simulink model "Example_PHEX"  (R2017a)
settings: Solver=VariableStepAuto  StartTime=0.0  StopTime=10.0  RelTol=1e-3
values from neighbouring files (symbols this model uses):
  L = [0.519243383422 0.571231761788 0.460093985593 1.39194595515 0.630156881592 0.260948993381 9.53677639553 0.00918592125768 0.177711077409 0.0643194958333 0.141274848846 0.223226056913 ... (18 elements, 9x2)]    [Example_PHEX.mat]
  u0 = [60 10 0.25 0.15]    [Example_PHEX.mat]
  x0 = [54.5367745473 47.8290809093 39.5934416646 44.0109305589 34.9055548044 23.7260654078 44.0109305589 39.5934416646 39.5934416646]    [Example_PHEX.mat]
  y0 = [44.0109305589 39.5934416646]    [Example_PHEX.mat]
undefined symbols (not defined in the file or in its folder): PHEX_sys_bilin
settings Model: Creator=lerch  LastModifiedBy=lerch
settings OptimizationCC: DefaultParameterBehavior=Inlined

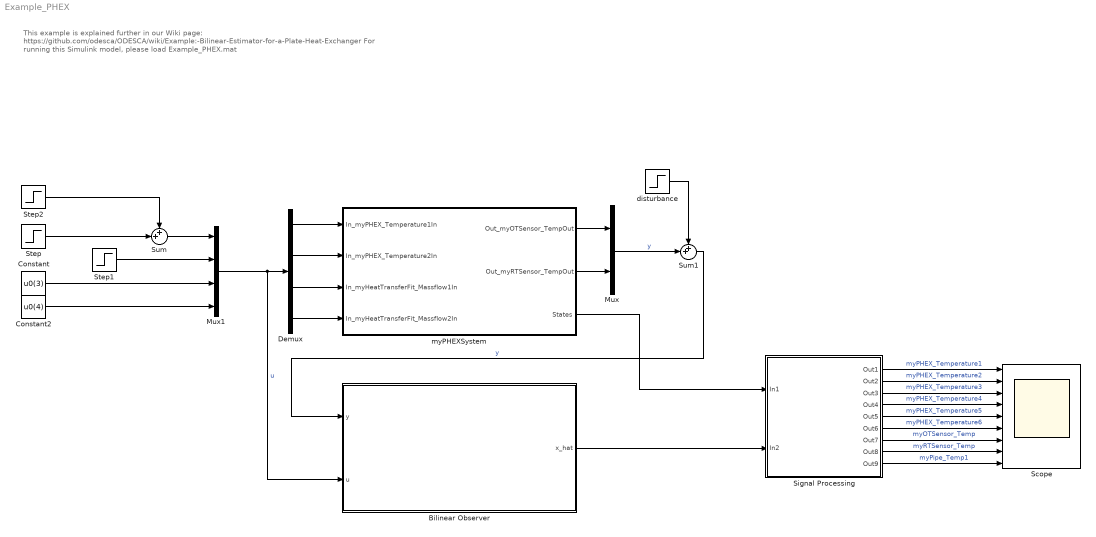
== system Example_PHEX ==
  note: This example is explained further in our Wiki page:
      | https://github.com/odesca/ODESCA/wiki/Example:-Bilinear-Estimator-for-a-Plate-Heat-Exchanger
      |
      | For running this Simulink model, please load Example_PHEX.mat
  Bilinear Observer : Subsystem
  Constant : Constant  Value=u0(3)
  Constant2 : Constant  Value=u0(4)
  Demux : Demux
  Mux : Mux  Inputs=2
  Mux1 : Mux
  Scope : Scope  NumInputPorts=9
  Signal Processing : Subsystem
  Step : Step  Before=u0(1)  After=u0(1)+20  SampleTime=0
  Step1 : Step  Time=3  Before=u0(2)  After=u0(2)+20  SampleTime=0
  Step2 : Step  Time=5  After=-40  SampleTime=0
  Sum : Sum  Inputs=++|
  Sum1 : Sum  Inputs=++|
  disturbance : Step  Time=7  After=5  SampleTime=0
  myPHEXSystem : Subsystem  mask(myPHEXSystem){initState=[0,0,0,0,0,0,0,0,0], myPHEX_cHex=500, myPHEX_mHex=1.154, myPHEX_Volume1=0.000216, myPHEX_Volume2=0.00024, myPHEX_HexArea=0.216, myPHEX_RhoFluid=998, myPHEX_cFluid=4182, myHeatTransferFit_c1=6529, myHeatTransferFit_c2=4029, myHeatTransferFit_c3=3.29, myOTSensor_TimeConst=1.8, myOTSensor_Gain=1, myPipe_cPipe=1, myPipe_mPipe=150, myPipe_VPipe=0.00055}
      mask prompts: initState "Initial State is a column vector of 9 elements:

x1 = myPHEX_Temperature1 [°C]
x2 = myPHEX_Temperature2 [°C]
x3 = myPHEX_Temperature3 [°C]
x4 = myPHEX_Temperature4 [°C]
x5 = myPHEX_Temperature5 [°C]
x6 = myPHEX_Temperature6 [°C]
x7 = myOTSensor_Temp [°C]
x8 = myRTSensor_Temp [°C]
x9 = myPipe_Temp1 [°C]

Initial State:"; myPHEX_cHex "cHex
[J/kg*K]"; myPHEX_mHex "mHex
[kg]"; myPHEX_Volume1 "Volume1
[m^3]"; myPHEX_Volume2 "Volume2
[m^3]"; myPHEX_HexArea "HexArea
[m^2]"; myPHEX_RhoFluid "RhoFluid
[kg/m^3]"; myPHEX_cFluid "cFluid
[J/kg*K]"; myHeatTransferFit_c1 "c1
[W/m^2*K)]"; myHeatTransferFit_c2 "c2
[W*s/m^2*K*kg]"; myHeatTransferFit_c3 "c3
[W*s/m^2*K*kg]"; myOTSensor_TimeConst "TimeConst
[s]"; myOTSensor_Gain "Gain
[1]"; myPipe_cPipe "cPipe
[J/kg*K]"; myPipe_mPipe "mPipe
[kg]"; myPipe_VPipe "VPipe
[m^3]"
      mask help:
      | This system consists of:
      |
      | 5 Components
      | 9 States
      | 4 Inputs
      | 2 Outputs
      | 15 Parameters
  wires:
  myPHEXSystem/1(Out_myOTSensor_TempOut) -> Mux/1
  myPHEXSystem/2(Out_myRTSensor_TempOut) -> Mux/2
  Sum1/1 -> Bilinear Observer/1(y)  "y"
  Demux/1 -> myPHEXSystem/1(In_myPHEX_Temperature1In)
  Demux/3 -> myPHEXSystem/3(In_myHeatTransferFit_Massflow1In)
  Demux/2 -> myPHEXSystem/2(In_myPHEX_Temperature2In)
  Demux/4 -> myPHEXSystem/4(In_myHeatTransferFit_Massflow2In)
  Mux1/1 -> Bilinear Observer/2(u), Demux/1  "u"
  myPHEXSystem/3(States) -> Signal Processing/1(In1)
  Bilinear Observer/1(x_hat) -> Signal Processing/2(In2)
  Signal Processing/1(Out1) -> Scope/1  "myPHEX_Temperature1"
  Signal Processing/2(Out2) -> Scope/2  "myPHEX_Temperature2"
  Signal Processing/3(Out3) -> Scope/3  "myPHEX_Temperature3"
  Signal Processing/4(Out4) -> Scope/4  "myPHEX_Temperature4"
  Signal Processing/5(Out5) -> Scope/5  "myPHEX_Temperature5"
  Signal Processing/6(Out6) -> Scope/6  "myPHEX_Temperature6"
  Signal Processing/7(Out7) -> Scope/7  "myOTSensor_Temp"
  Signal Processing/8(Out8) -> Scope/8  "myRTSensor_Temp"
  Signal Processing/9(Out9) -> Scope/9  "myPipe_Temp1"
  Step/1 -> Sum/2
  Step1/1 -> Mux1/2
  Constant/1 -> Mux1/3
  Constant2/1 -> Mux1/4
  Sum/1 -> Mux1/1
  Step2/1 -> Sum/1
  Mux/1 -> Sum1/2  "y"
  disturbance/1 -> Sum1/1

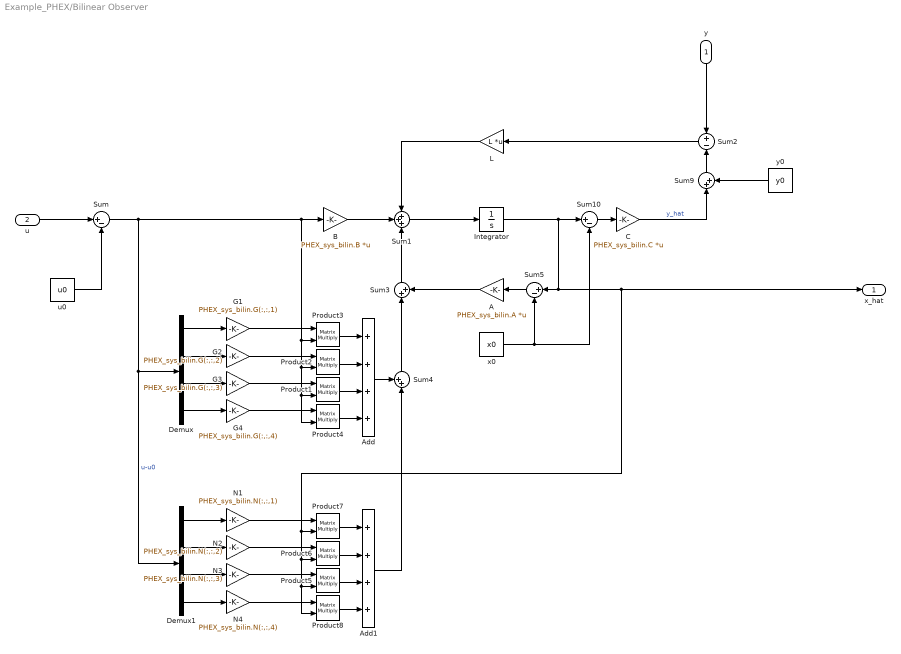
== system Example_PHEX/Bilinear Observer ==
  y : Inport
  u : Inport  Port=2
  A : Gain  Gain=PHEX_sys_bilin.A  Multiplication=Matrix(K*u) (u vector)
  Add : Sum  Inputs=++++
  Add1 : Sum  Inputs=++++
  B : Gain  Gain=PHEX_sys_bilin.B  Multiplication=Matrix(K*u) (u vector)
  C : Gain  Gain=PHEX_sys_bilin.C  Multiplication=Matrix(K*u) (u vector)
  Demux : Demux
  Demux1 : Demux
  G1 : Gain  Gain=PHEX_sys_bilin.G(:,:,1)
  G2 : Gain  Gain=PHEX_sys_bilin.G(:,:,2)
  G3 : Gain  Gain=PHEX_sys_bilin.G(:,:,3)
  G4 : Gain  Gain=PHEX_sys_bilin.G(:,:,4)
  Integrator : Integrator
  L : Gain  Gain=L  Multiplication=Matrix(K*u) (u vector)
  N1 : Gain  Gain=PHEX_sys_bilin.N(:,:,1)
  N2 : Gain  Gain=PHEX_sys_bilin.N(:,:,2)
  N3 : Gain  Gain=PHEX_sys_bilin.N(:,:,3)
  N4 : Gain  Gain=PHEX_sys_bilin.N(:,:,4)
  Product{1..8} (8 alike) : Product  Multiplication=Matrix(*)
  Sum : Sum  Inputs=|+-
  Sum1 : Sum  Inputs=+++
  Sum10 : Sum  Inputs=|+-
  Sum2 : Sum  Inputs=+-
  Sum3 : Sum  Inputs=|++
  Sum4 : Sum  Inputs=++|
  Sum5 : Sum  Inputs=|+-
  Sum9 : Sum  Inputs=|++
  u0 : Constant  Value=u0
  x0 : Constant  Value=x0
  "y0 " : Constant  Value=y0
  x_hat : Outport
  wires:
  u/1 -> Sum/1
  u0/1 -> Sum/2
  B/1 -> Sum1/2
  Sum1/1 -> Integrator/1
  C/1 -> Sum9/1  "y_hat"
  L/1 -> Sum1/1
  Sum2/1 -> L/1
  Sum5/1 -> A/1
  x0/1 -> Sum5/2, Sum10/2
  Sum10/1 -> C/1
  y/1 -> Sum2/1
  Sum9/1 -> Sum2/2
  "y0 "/1 -> Sum9/2
  Sum3/1 -> Sum1/3
  A/1 -> Sum3/2
  Demux/1 -> G1/1
  Demux/2 -> G2/1
  Demux/3 -> G3/1
  Demux/4 -> G4/1
  G1/1 -> Product3/1
  G2/1 -> Product2/1
  G3/1 -> Product1/1
  G4/1 -> Product4/1
  Product3/1 -> Add/1
  Product2/1 -> Add/2
  Product1/1 -> Add/3
  Product4/1 -> Add/4
  Add/1 -> Sum4/1
  Sum4/1 -> Sum3/1
  Add1/1 -> Sum4/2
  Product8/1 -> Add1/4
  Product5/1 -> Add1/3
  Product6/1 -> Add1/2
  Product7/1 -> Add1/1
  N4/1 -> Product8/1
  N3/1 -> Product5/1
  N2/1 -> Product6/1
  N1/1 -> Product7/1
  Demux1/4 -> N4/1
  Demux1/3 -> N3/1
  Demux1/2 -> N2/1
  Demux1/1 -> N1/1
  Integrator/1 -> Sum10/1, Sum5/1, Product7/2, Product6/2, Product5/2, Product8/2, x_hat/1
  Sum/1 -> Demux1/1, Demux/1, Product4/2, Product1/2, Product2/2, Product3/2, B/1  "u-u0"

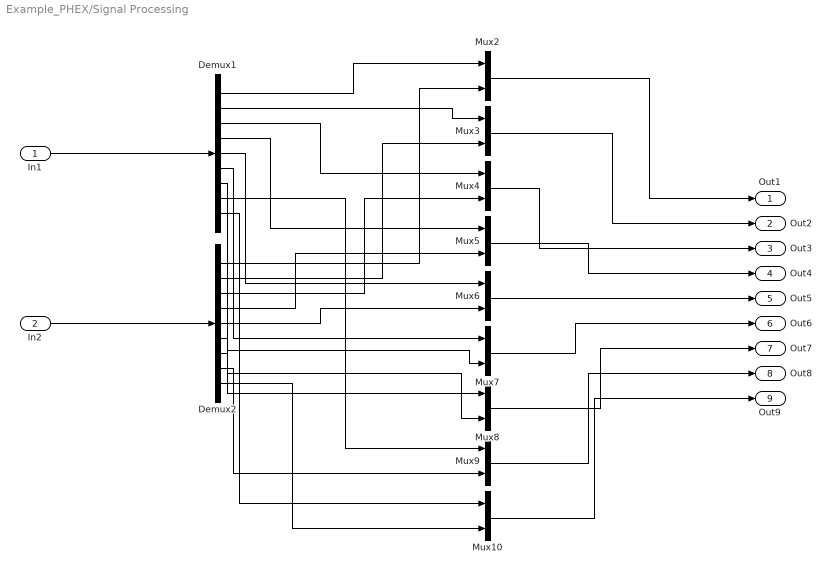
== system Example_PHEX/Signal Processing ==
  In1 : Inport
  In2 : Inport  Port=2
  Demux1 : Demux  Outputs=9
  Demux2 : Demux  Outputs=9
  Mux{2..10} (9 alike) : Mux  Inputs=2
  Out1 : Outport
  Out2 : Outport  Port=2
  Out3 : Outport  Port=3
  Out4 : Outport  Port=4
  Out5 : Outport  Port=5
  Out6 : Outport  Port=6
  Out7 : Outport  Port=7
  Out8 : Outport  Port=8
  Out9 : Outport  Port=9
  wires:
  Demux1/6 -> Mux7/1
  Demux1/4 -> Mux5/1
  In2/1 -> Demux2/1
  Demux2/8 -> Mux9/2
  Demux1/9 -> Mux10/1
  Demux1/8 -> Mux9/1
  Demux2/1 -> Mux2/2
  Demux1/7 -> Mux8/1
  Demux1/2 -> Mux3/1
  Demux1/3 -> Mux4/1
  Demux1/1 -> Mux2/1
  In1/1 -> Demux1/1
  Demux2/4 -> Mux5/2
  Mux7/1 -> Out6/1
  Demux1/5 -> Mux6/1
  Demux2/2 -> Mux3/2
  Demux2/7 -> Mux8/2
  Demux2/5 -> Mux6/2
  Demux2/9 -> Mux10/2
  Demux2/6 -> Mux7/2
  Demux2/3 -> Mux4/2
  Mux2/1 -> Out1/1
  Mux3/1 -> Out2/1
  Mux5/1 -> Out4/1
  Mux6/1 -> Out5/1
  Mux4/1 -> Out3/1
  Mux10/1 -> Out9/1
  Mux8/1 -> Out7/1
  Mux9/1 -> Out8/1

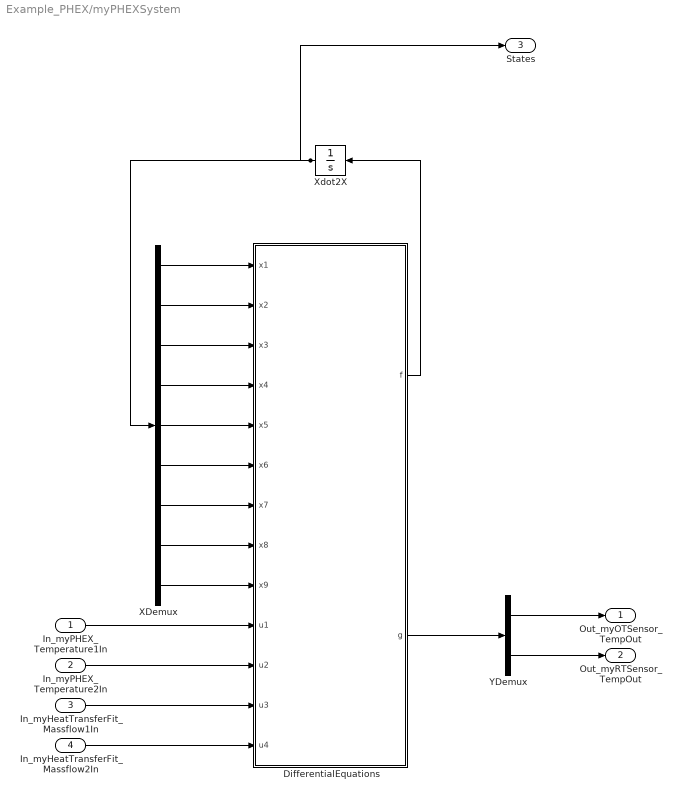
== system Example_PHEX/myPHEXSystem ==
  In_myPHEX_Temperature1In : Inport
  In_myPHEX_Temperature2In : Inport  Port=2
  In_myHeatTransferFit_Massflow1In : Inport  Port=3
  In_myHeatTransferFit_Massflow2In : Inport  Port=4
  DifferentialEquations : MATLAB Function  TreatAsAtomicUnit=on
  XDemux : Demux  Outputs=9
  Xdot2X : Integrator  InitialCondition=initState
  YDemux : Demux  Outputs=2
  Out_myOTSensor_TempOut : Outport
  Out_myRTSensor_TempOut : Outport  Port=2
  States : Outport  Port=3
  wires:
  In_myPHEX_Temperature1In/1 -> DifferentialEquations/10(u1)
  In_myPHEX_Temperature2In/1 -> DifferentialEquations/11(u2)
  In_myHeatTransferFit_Massflow1In/1 -> DifferentialEquations/12(u3)
  In_myHeatTransferFit_Massflow2In/1 -> DifferentialEquations/13(u4)
  DifferentialEquations/2(g) -> YDemux/1
  YDemux/1 -> Out_myOTSensor_TempOut/1
  YDemux/2 -> Out_myRTSensor_TempOut/1
  XDemux/1 -> DifferentialEquations/1(x1)
  XDemux/2 -> DifferentialEquations/2(x2)
  XDemux/3 -> DifferentialEquations/3(x3)
  XDemux/4 -> DifferentialEquations/4(x4)
  XDemux/5 -> DifferentialEquations/5(x5)
  XDemux/6 -> DifferentialEquations/6(x6)
  XDemux/7 -> DifferentialEquations/7(x7)
  XDemux/8 -> DifferentialEquations/8(x8)
  XDemux/9 -> DifferentialEquations/9(x9)
  DifferentialEquations/1(f) -> Xdot2X/1
  Xdot2X/1 -> XDemux/1, States/1

== matlab function Example_PHEX/myPHEXSystem/DifferentialEquations ==
  data: x1 input; f output; x2 input; x3 input; x4 input; x5 input; x6 input; x7 input; x8 input; x9 input; u1 input; u2 input; u3 input; u4 input; g output; myPipe_VPipe parameter; myPipe_mPipe parameter; myPipe_cPipe parameter; myOTSensor_Gain parameter; myOTSensor_TimeConst parameter; myHeatTransferFit_c3 parameter; myHeatTransferFit_c2 parameter; myHeatTransferFit_c1 parameter; myPHEX_cFluid parameter; myPHEX_RhoFluid parameter; myPHEX_HexArea parameter; myPHEX_Volume2 parameter; myPHEX_Volume1 parameter; myPHEX_mHex parameter; myPHEX_cHex parameter
function [f,g] = DifferentialEquations(x1,x2,x3,x4,x5,x6,x7,x8,x9,u1,u2,u3,u4,myPipe_VPipe, myPipe_mPipe, myPipe_cPipe, myOTSensor_Gain, myOTSensor_TimeConst, myHeatTransferFit_c3, myHeatTransferFit_c2, myHeatTransferFit_c1, myPHEX_cFluid, myPHEX_RhoFluid, myPHEX_HexArea, myPHEX_Volume2, myPHEX_Volume1, myPHEX_mHex, myPHEX_cHex)
%#codegen

%    This function was generated by the Symbolic Math Toolbox version 7.2.
%    02-Jul-2019 09:48:33

t2 = myHeatTransferFit_c2.*u3;
t3 = myHeatTransferFit_c3.*u4;
t4 = myHeatTransferFit_c1+t2+t3;
t5 = myPHEX_cHex.*myPHEX_mHex.*(1.0./6.0);
t6 = myPHEX_cFluid.*myPHEX_Volume1.*myPHEX_RhoFluid.*(1.0./3.0);
t7 = t5+t6;
t8 = 1.0./t7;
t9 = x1-x4;
t10 = myPHEX_HexArea.*t4.*t9.*(1.0./3.0);
t11 = x2-x5;
t12 = myPHEX_HexArea.*t4.*t11.*(1.0./3.0);
t13 = myPHEX_cFluid.*myPHEX_Volume2.*myPHEX_RhoFluid.*(1.0./3.0);
t14 = t5+t13;
t15 = 1.0./t14;
t16 = x3-x6;
t17 = myPHEX_HexArea.*t4.*t16.*(1.0./3.0);
t18 = 1.0./myOTSensor_TimeConst;
f = [-t8.*(t10-myPHEX_cFluid.*u3.*(u1-x1));-t8.*(t12-myPHEX_cFluid.*u3.*(x1-x2));-t8.*(t17-myPHEX_cFluid.*u3.*(x2-x3));t15.*(t10-myPHEX_cFluid.*u4.*(x4-x5));t15.*(t12-myPHEX_cFluid.*u4.*(x5-x6));t15.*(t17+myPHEX_cFluid.*u4.*(u2-x6));-t18.*(x7-myOTSensor_Gain.*x4);-t18.*(x8-myOTSensor_Gain.*x9);(myPHEX_cFluid.*u3.*(x3-x9))./(myPipe_cPipe.*myPipe_mPipe+myPipe_VPipe.*myPHEX_cFluid.*myPHEX_RhoFluid)];
if nargout > 1
    g = [x7;x8];
end
